simulink model "ex2busStability_sim"  (R2014b)
settings: Solver=ode45  SolverMode=SingleTasking  StartTime=0  StopTime=10  MaxStep=0.001  RelTol=1e-06
values from neighbouring files (symbols this model uses):
  A = full(A)    [ex3busPV.m]
  B = full(B)    [ex3busPV.m]
  C = full(C)    [ex3busPV.m]    (also in ex_get_started_here.m = 5e-07; pv_dq.m = 4.01652892562e-06)
  cur_dq0_op = 2^0.5*[-iopx; iopx; -iopy; iopy; 0; 0]    [ex2busStability.m]
  D = full(D)    [ex3busPV.m]
  Kd = KD_GAIN_CNST*J*ws    [ex14busSGandPV.m]    (also in ex2busStability.m = 24000; ex7busLongLine.m; ex9busSG.m; exDroopA.m)
  lamda = (2^0.5) * Vgmag/ws    (= 45.916132124)    [ex2busStability.m]    (also in ex9busSG.m = (2^0.5) * Vn_gens/ws)
  Pm_op = 3*Pg    (= 600000)    [ex2busStability.m]
  poles_2Jws = poles./(2*J*ws)    [ex14busSGandPV.m]    (also in ex2busStability.m = poles./(2*ws*J); ex7busLongLine.m; ex9busSG.m = poles./(2*ws*J); exDroopA.m)
  step_size = 30e3    (= 30000)    [ex2busStability.m]    (also in exDroopB.m = 0)
  step_time = 9    [ex2busStability.m]    (also in ex3busPV.m = 0.05; exDroopB.m = 10; exLongLinePV.m = 1; syncMachVsSwing.m = 5)
  V1mag = 10e3    (= 10000)    [ex2busStability.m]
  vol_dq0_op = 2^0.5*[V1mag; vopx; 0; vopy; 0; 0]    [ex2busStability.m]
  ws = 2*pi*50    (= 314.159265359)    [ex14busSGandPV.m]    (also in ex2busStability.m; ex3busPV.m; ex7busLongLine.m; ex9busSG.m)
undefined symbols (not defined in the file or in its folder): Anet, Bnet, Cnet, Dnet, full
settings Model: Creator=COPEC  LastModifiedBy=Juri
settings OptimizationCC: BlockReduction=off  BooleanDataType=off
settings DebuggingCC: SaveWithParameterizedLinksMsg=none  UnderspecifiedInitializationDetection=Classic  MergeDetectMultiDrivingBlocksExec=none  SignalResolutionControl=TryResolveAllWithWarning  SolverPrmCheckMsg=none  FrameProcessingCompatibilityMsg=error
settings HardwareCC: TargetUnknown=on

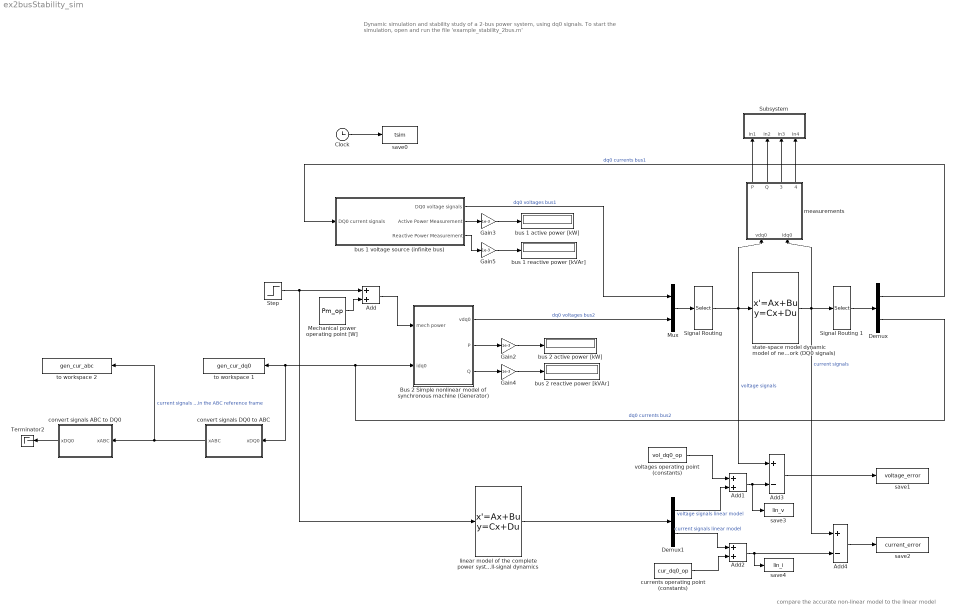
== system ex2busStability_sim ==
  note: Dynamic simulation and stability study of a 2-bus power system,
      | using dq0 signals.
      |
      | To start the simulation, open and run the file
      | 'example_stability_2bus.m'
  note: compare the accurate non-linear model to the linear model
  Add : Sum
  Add1 : Sum
  Add2 : Sum
  Add3 : Sum  Inputs=+-
  Add4 : Sum  Inputs=+-
  Bus 2 Simple nonlinear model of synchronous machine (Generator) : Subsystem
  Clock : Clock
  Demux : Demux  Outputs=2
  Demux1 : Demux  Outputs=2
  Gain{2..5} (4 alike) : Gain  Gain=1e-3
  Mechanical power operating point [W] : Constant  Value=Pm_op
  Mux : Mux  Inputs=2
  "Signal Routing " : Selector  InputPortWidth=6  IndexOptions=Index vector (dialog)  Indices=[1 4 2 5 3 6]  OutputSizes=1
  Signal Routing 1 : Selector  InputPortWidth=6  IndexOptions=Index vector (dialog)  Indices=[1 3 5 2 4 6]  OutputSizes=1
  Step : Step  Time=step_time  After=step_size  SampleTime=0
  Subsystem : Subsystem
  Terminator2 : Terminator
  bus 1 voltage source (infinite bus) : Subsystem
  bus 1 active power [kW] : Display
  bus 1 reactive power [kVAr] : Display
  bus 2 active power [kW] : Display
  bus 2 reactive power [kVAr] : Display
  convert signals ABC to DQ0 : Subsystem
  convert signals DQ0 to ABC : Subsystem
  currents operating point (constants) : Constant  Value=cur_dq0_op
  "linear model of the complete power system (network + generator) this state-space model represents the system small-signal dynamics " : StateSpace  A=full(A)  B=full(B)  C=full(C)  D=full(D)  X0=0
  measurements : Subsystem
  save0 : ToWorkspace  VariableName=tsim  SampleTime=-1
  save1 : ToWorkspace  VariableName=voltage_error  SampleTime=-1
  save2 : ToWorkspace  VariableName=current_error  SampleTime=-1
  save3 : ToWorkspace  VariableName=lin_v  SampleTime=-1
  save4 : ToWorkspace  VariableName=lin_i  SampleTime=-1
  state-space model dynamic model of network (DQ0 signals) : StateSpace  A=full(Anet)  B=full(Bnet)  C=full(Cnet)  D=full(Dnet)  X0=0
  to workspace 1 : ToWorkspace  VariableName=gen_cur_dq0  SampleTime=-1
  to workspace 2 : ToWorkspace  VariableName=gen_cur_abc  SampleTime=-1
  voltages operating point (constants) : Constant  Value=vol_dq0_op
  wires:
  Clock/1 -> save0/1
  Gain2/1 -> bus 2 active power [kW]/1
  Gain4/1 -> bus 2 reactive power [kVAr]/1
  Mechanical power operating point [W]/1 -> Add/2
  Mux/1 -> "Signal Routing "/1
  Signal Routing 1/1 -> Demux/1
  Bus 2 Simple nonlinear model of synchronous machine (Generator)/2(P) -> Gain2/1
  Bus 2 Simple nonlinear model of synchronous machine (Generator)/3(Q) -> Gain4/1
  "Signal Routing "/1 -> Add3/1, state-space model dynamic model of network (DQ0 signals)/1, measurements/1(vdq0)  "voltage signals"
  bus 1 voltage source (infinite bus)/1(DQ0 voltage signals) -> Mux/1  "dq0 voltages bus1"
  Bus 2 Simple nonlinear model of synchronous machine (Generator)/1(vdq0) -> Mux/2  "dq0 voltages bus2"
  Demux/1 -> bus 1 voltage source (infinite bus)/1(DQ0 current signals)  "dq0 currents bus1"
  Demux/2 -> to workspace 1/1, convert signals DQ0 to ABC/1(xDQ0), Bus 2 Simple nonlinear model of synchronous machine (Generator)/2(idq0)  "dq0 currents bus2"
  state-space model dynamic model of network (DQ0 signals)/1 -> Add4/1, measurements/2(idq0), Signal Routing 1/1  "current signals"
  convert signals DQ0 to ABC/1(xABC) -> to workspace 2/1, convert signals ABC to DQ0/1(xABC)  "current signals in the ABC reference frame"
  convert signals ABC to DQ0/1(xDQ0) -> Terminator2/1
  bus 1 voltage source (infinite bus)/2(Active Power Measurement) -> Gain3/1
  bus 1 voltage source (infinite bus)/3("Reactive Power Measurement ") -> Gain5/1
  Gain3/1 -> bus 1 active power [kW]/1
  Gain5/1 -> bus 1 reactive power [kVAr]/1
  Add/1 -> Bus 2 Simple nonlinear model of synchronous machine (Generator)/1(mech power)
  Step/1 -> "linear model of the complete power system (network + generator) this state-space model represents the system small-signal dynamics "/1, Add/1
  "linear model of the complete power system (network + generator) this state-space model represents the system small-signal dynamics "/1 -> Demux1/1
  Demux1/1 -> Add1/2  "voltage signals linear model"
  Demux1/2 -> Add2/1  "current signals linear model"
  voltages operating point (constants)/1 -> Add1/1
  currents operating point (constants)/1 -> Add2/2
  Add1/1 -> save3/1, Add3/2
  Add2/1 -> save4/1, Add4/2
  Add3/1 -> save1/1
  Add4/1 -> save2/1
  measurements/1(P) -> Subsystem/1(In1)
  measurements/2(Q) -> Subsystem/2(In2)
  measurements/3(Vm_RMS) -> Subsystem/3(In3)
  measurements/4(Vph_deg) -> Subsystem/4(In4)

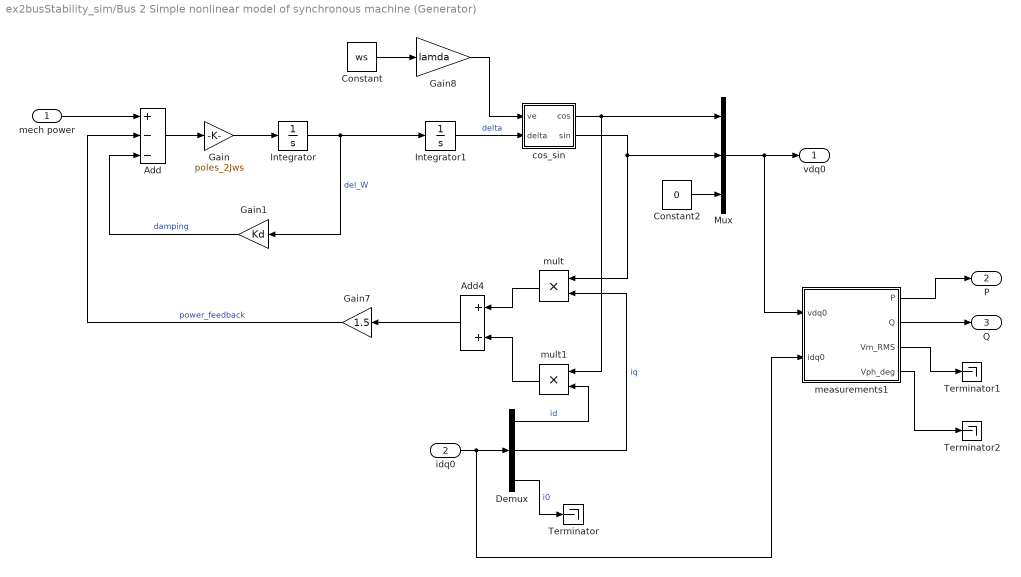
== system ex2busStability_sim/Bus 2 Simple nonlinear model of synchronous machine (Generator) ==
  mech power : Inport
  idq0 : Inport  Port=2
  Add : Sum  Inputs=+--
  Add4 : Sum
  Constant : Constant  Value=ws
  Constant2 : Constant  Value=0
  Demux : Demux  Outputs=3
  Gain : Gain  Gain=poles_2Jws
  Gain1 : Gain  Gain=Kd
  Gain7 : Gain  Gain=1.5
  Gain8 : Gain  Gain=lamda
  Integrator : Integrator
  Integrator1 : Integrator
  Mux : Mux  Inputs=3
  Terminator : Terminator
  Terminator1 : Terminator
  Terminator2 : Terminator
  cos_sin : Subsystem
  measurements1 : Subsystem
  mult : Product  Inputs=**
  mult1 : Product  Inputs=**
  vdq0 : Outport
  P : Outport  Port=2
  Q : Outport  Port=3
  wires:
  mech power/1 -> Add/1
  Add/1 -> Gain/1
  Gain/1 -> Integrator/1
  Integrator/1 -> Gain1/1, Integrator1/1  "del_W"
  Integrator1/1 -> cos_sin/2(delta)  "delta"
  Gain1/1 -> Add/3  "damping"
  Demux/3 -> Terminator/1  "i0"
  cos_sin/1(cos) -> mult1/1, Mux/1
  cos_sin/2(sin) -> mult/1, Mux/2
  mult/1 -> Add4/1
  mult1/1 -> Add4/2
  Add4/1 -> Gain7/1
  Gain7/1 -> Add/2  "power_feedback"
  idq0/1 -> measurements1/2(idq0), Demux/1
  Mux/1 -> measurements1/1(vdq0), vdq0/1
  Constant/1 -> Gain8/1
  Gain8/1 -> cos_sin/1(ve)
  Constant2/1 -> Mux/3
  Demux/1 -> mult1/2  "id"
  Demux/2 -> mult/2  "iq"
  measurements1/1(P) -> P/1
  measurements1/2(Q) -> Q/1
  measurements1/3(Vm_RMS) -> Terminator1/1
  measurements1/4(Vph_deg) -> Terminator2/1

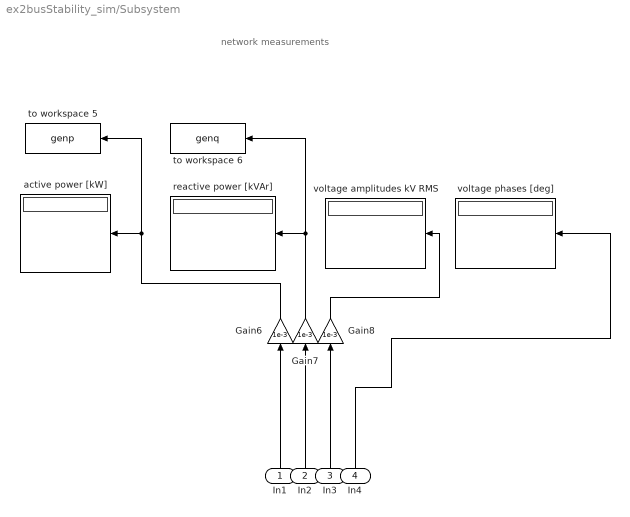
== system ex2busStability_sim/Subsystem ==
  note: network measurements
  In1 : Inport
  In2 : Inport  Port=2
  In3 : Inport  Port=3
  In4 : Inport  Port=4
  Gain6 : Gain  Gain=1e-3
  Gain7 : Gain  Gain=1e-3
  Gain8 : Gain  Gain=1e-3
  active power [kW] : Display
  reactive power [kVAr] : Display
  to workspace 5 : ToWorkspace  VariableName=genp  SampleTime=-1
  to workspace 6 : ToWorkspace  VariableName=genq  SampleTime=-1
  "voltage amplitudes kV RMS " : Display
  voltage phases [deg] : Display
  wires:
  Gain6/1 -> to workspace 5/1, active power [kW]/1
  In1/1 -> Gain6/1
  In3/1 -> Gain8/1
  In2/1 -> Gain7/1
  Gain8/1 -> "voltage amplitudes kV RMS "/1
  Gain7/1 -> to workspace 6/1, reactive power [kVAr]/1
  In4/1 -> voltage phases [deg]/1

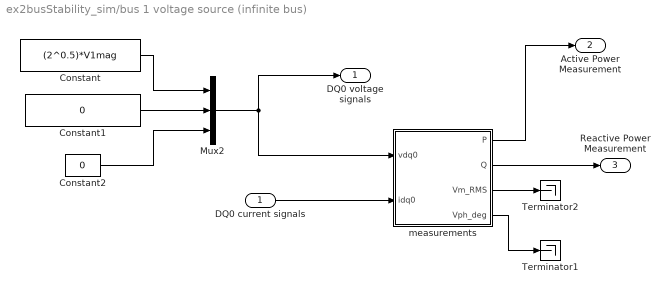
== system ex2busStability_sim/bus 1 voltage source (infinite bus) ==
  DQ0 current signals : Inport
  Constant : Constant  Value=(2^0.5)*V1mag
  Constant1 : Constant  Value=0
  Constant2 : Constant  Value=0
  Mux2 : Mux  Inputs=3
  Terminator1 : Terminator
  Terminator2 : Terminator
  measurements : Subsystem
  DQ0 voltage signals : Outport
  Active Power Measurement : Outport  Port=2
  "Reactive Power Measurement " : Outport  Port=3
  wires:
  Constant/1 -> Mux2/1
  Constant1/1 -> Mux2/2
  Constant2/1 -> Mux2/3
  Mux2/1 -> measurements/1(vdq0), DQ0 voltage signals/1
  DQ0 current signals/1 -> measurements/2(idq0)
  measurements/1(P) -> Active Power Measurement/1
  measurements/2(Q) -> "Reactive Power Measurement "/1
  measurements/3(Vm_RMS) -> Terminator2/1
  measurements/4(Vph_deg) -> Terminator1/1

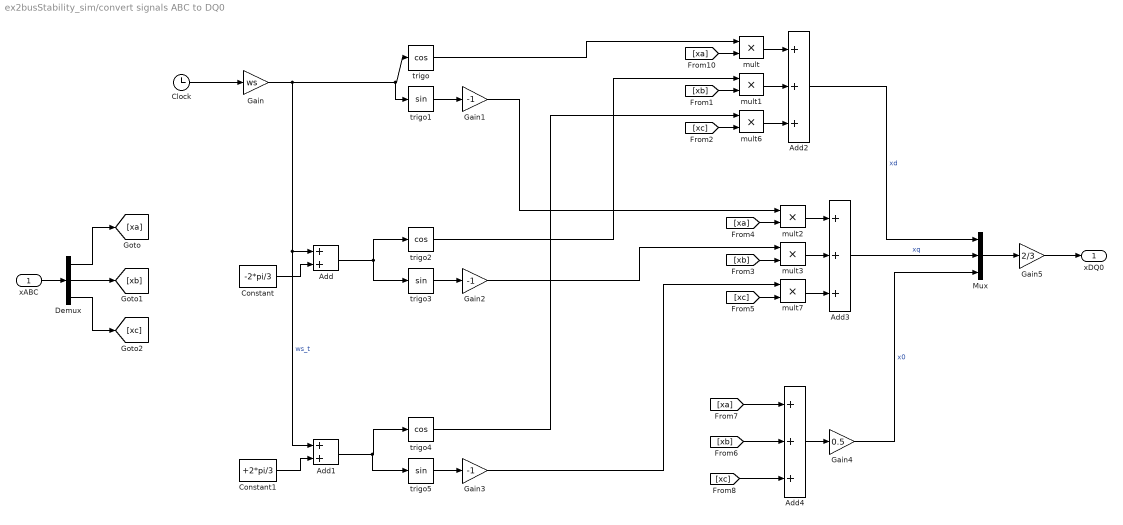
== system ex2busStability_sim/convert signals ABC to DQ0 ==
  xABC : Inport
  Add : Sum
  Add1 : Sum
  Add2 : Sum  Inputs=+++
  Add3 : Sum  Inputs=+++
  Add4 : Sum  Inputs=+++
  Clock : Clock
  Constant : Constant  Value=-2*pi/3
  Constant1 : Constant  Value=+2*pi/3
  Demux : Demux  Outputs=3
  Gain : Gain  Gain=ws
  Gain1 : Gain  Gain=-1
  Gain2 : Gain  Gain=-1
  Gain3 : Gain  Gain=-1
  Gain4 : Gain  Gain=0.5
  Gain5 : Gain  Gain=2/3
  Mux : Mux  Inputs=3
  mult{,1..3,6..7} (6 alike) : Product  Inputs=**
  trigo : Trigonometry  Operator=cos
  trigo1 : Trigonometry
  trigo2 : Trigonometry  Operator=cos
  trigo3 : Trigonometry
  trigo4 : Trigonometry  Operator=cos
  trigo5 : Trigonometry
  xDQ0 : Outport
  wires:
  Gain5/1 -> xDQ0/1
  Mux/1 -> Gain5/1
  Gain3/1 -> mult7/1
  Gain2/1 -> mult3/1
  Gain1/1 -> mult2/1
  [xc] -> Add4/3
  [xb] -> Add4/2
  [xa] -> Add4/1
  Add4/1 -> Gain4/1
  mult7/1 -> Add3/3
  [xc] -> mult7/2
  [xb] -> mult3/2
  [xa] -> mult2/2
  trigo4/1 -> mult6/1
  mult6/1 -> Add2/3
  [xc] -> mult6/2
  trigo2/1 -> mult1/1
  trigo/1 -> mult/1
  Gain4/1 -> Mux/3  "x0"
  Add3/1 -> Mux/2  "xq"
  Add2/1 -> Mux/1  "xd"
  mult3/1 -> Add3/2
  mult2/1 -> Add3/1
  [xb] -> mult1/2
  [xa] -> mult/2
  mult1/1 -> Add2/2
  mult/1 -> Add2/1
  Demux/3 -> [xc]
  Demux/2 -> [xb]
  Demux/1 -> [xa]
  xABC/1 -> Demux/1
  Add1/1 -> trigo4/1, trigo5/1
  trigo5/1 -> Gain3/1
  Add/1 -> trigo3/1, trigo2/1
  trigo3/1 -> Gain2/1
  trigo1/1 -> Gain1/1
  Constant1/1 -> Add1/2
  Constant/1 -> Add/2
  Gain/1 -> Add/1, Add1/1, trigo/1, trigo1/1  "ws_t"
  Clock/1 -> Gain/1

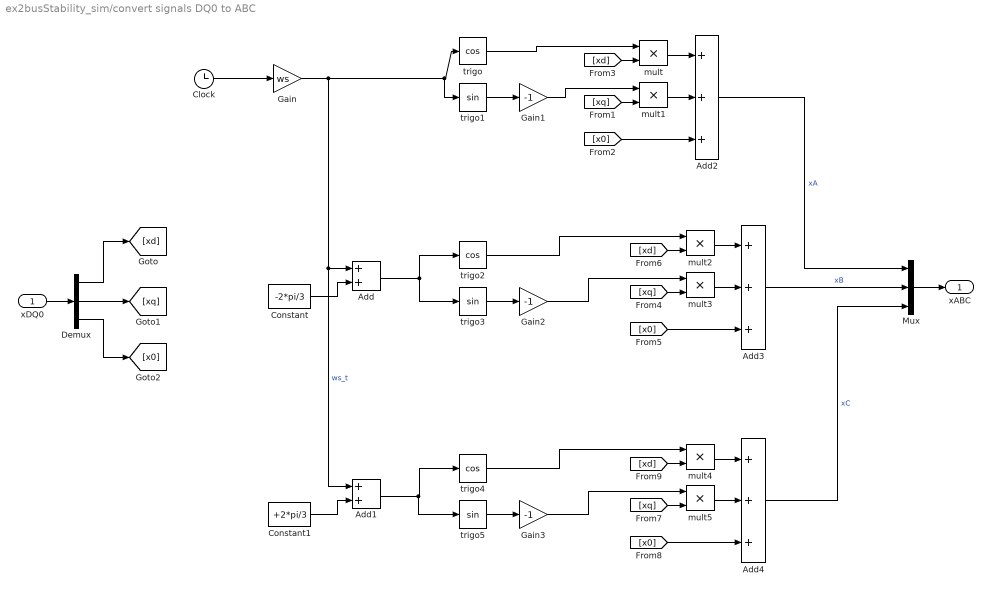
== system ex2busStability_sim/convert signals DQ0 to ABC ==
  xDQ0 : Inport
  Add : Sum
  Add1 : Sum
  Add2 : Sum  Inputs=+++
  Add3 : Sum  Inputs=+++
  Add4 : Sum  Inputs=+++
  Clock : Clock
  Constant : Constant  Value=-2*pi/3
  Constant1 : Constant  Value=+2*pi/3
  Demux : Demux  Outputs=3
  Gain : Gain  Gain=ws
  Gain1 : Gain  Gain=-1
  Gain2 : Gain  Gain=-1
  Gain3 : Gain  Gain=-1
  Mux : Mux  Inputs=3
  mult{,1..5} (6 alike) : Product  Inputs=**
  trigo : Trigonometry  Operator=cos
  trigo1 : Trigonometry
  trigo2 : Trigonometry  Operator=cos
  trigo3 : Trigonometry
  trigo4 : Trigonometry  Operator=cos
  trigo5 : Trigonometry
  xABC : Outport
  wires:
  Clock/1 -> Gain/1
  Gain/1 -> trigo1/1, trigo/1, Add1/1, Add/1  "ws_t"
  Constant/1 -> Add/2
  Constant1/1 -> Add1/2
  trigo1/1 -> Gain1/1
  trigo3/1 -> Gain2/1
  Add/1 -> trigo2/1, trigo3/1
  trigo5/1 -> Gain3/1
  Add1/1 -> trigo5/1, trigo4/1
  xDQ0/1 -> Demux/1
  Demux/1 -> [xd]
  Demux/2 -> [xq]
  Demux/3 -> [x0]
  Mux/1 -> xABC/1
  mult/1 -> Add2/1
  mult1/1 -> Add2/2
  [xd] -> mult/2
  [xq] -> mult1/2
  [x0] -> Add2/3
  mult2/1 -> Add3/1
  mult3/1 -> Add3/2
  [xd] -> mult2/2
  [xq] -> mult3/2
  [x0] -> Add3/3
  mult4/1 -> Add4/1
  mult5/1 -> Add4/2
  [xd] -> mult4/2
  [xq] -> mult5/2
  [x0] -> Add4/3
  trigo/1 -> mult/1
  Gain1/1 -> mult1/1
  trigo2/1 -> mult2/1
  Gain2/1 -> mult3/1
  trigo4/1 -> mult4/1
  Gain3/1 -> mult5/1
  Add2/1 -> Mux/1  "xA"
  Add3/1 -> Mux/2  "xB"
  Add4/1 -> Mux/3  "xC"

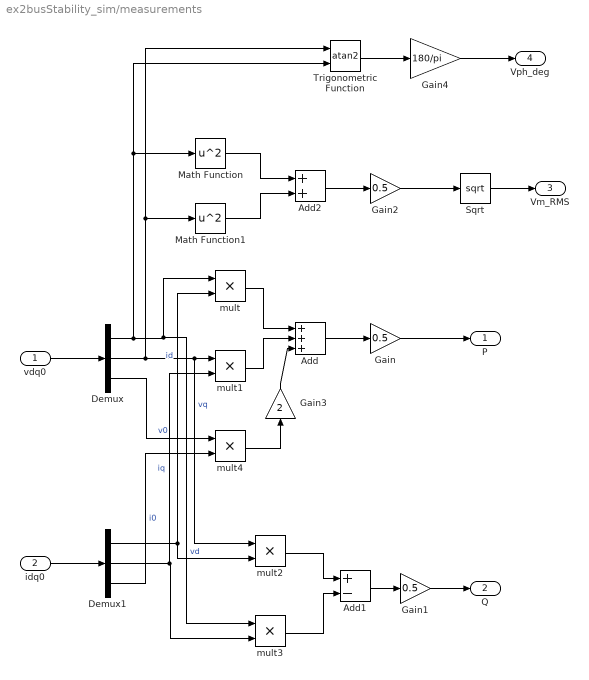
== system ex2busStability_sim/measurements ==
  vdq0 : Inport
  idq0 : Inport  Port=2
  Add : Sum  Inputs=+++
  Add1 : Sum  Inputs=+-
  Add2 : Sum
  Demux : Demux  Outputs=3
  Demux1 : Demux  Outputs=3
  Gain : Gain  Gain=0.5
  Gain1 : Gain  Gain=0.5
  Gain2 : Gain  Gain=0.5
  Gain3 : Gain  Gain=2
  Gain4 : Gain  Gain=180/pi
  Math Function : Math  Operator=square  SaturateOnIntegerOverflow=on
  Math Function1 : Math  Operator=square  SaturateOnIntegerOverflow=on
  Sqrt : Sqrt  SaturateOnIntegerOverflow=on
  Trigonometric Function : Trigonometry  Operator=atan2
  mult{,1..4} (5 alike) : Product  Inputs=**
  P : Outport
  Q : Outport  Port=2
  Vm_RMS : Outport  Port=3
  Vph_deg : Outport  Port=4
  wires:
  idq0/1 -> Demux1/1
  vdq0/1 -> Demux/1
  Demux/1 -> Math Function/1, Trigonometric Function/2, mult3/1, mult/1  "vd"
  Demux/2 -> Trigonometric Function/1, Math Function1/1, mult2/1, mult1/1  "vq"
  Demux1/1 -> mult/2, mult2/2  "id"
  Demux1/2 -> mult3/2, mult1/2  "iq"
  Demux/3 -> mult4/1  "v0"
  Demux1/3 -> mult4/2  "i0"
  mult/1 -> Add/1
  mult1/1 -> Add/2
  Add/1 -> Gain/1
  mult2/1 -> Add1/1
  mult3/1 -> Add1/2
  Add1/1 -> Gain1/1
  Sqrt/1 -> Vm_RMS/1
  Math Function/1 -> Add2/1
  Math Function1/1 -> Add2/2
  Add2/1 -> Gain2/1
  Gain2/1 -> Sqrt/1
  Gain/1 -> P/1
  Gain1/1 -> Q/1
  mult4/1 -> Gain3/1
  Gain3/1 -> Add/3
  Trigonometric Function/1 -> Gain4/1
  Gain4/1 -> Vph_deg/1

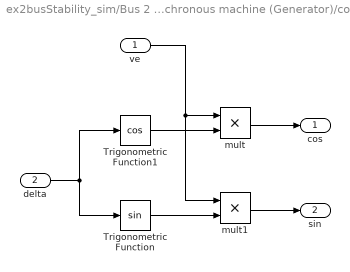
== system ex2busStability_sim/Bus 2 Simple nonlinear model of synchronous machine (Generator)/cos_sin ==
  ve : Inport
  delta : Inport  Port=2
  Trigonometric Function : Trigonometry
  Trigonometric Function1 : Trigonometry  Operator=cos
  mult : Product  Inputs=**
  mult1 : Product  Inputs=**
  cos : Outport
  sin : Outport  Port=2
  wires:
  delta/1 -> Trigonometric Function/1, Trigonometric Function1/1
  Trigonometric Function1/1 -> mult/2
  ve/1 -> mult1/1, mult/1
  Trigonometric Function/1 -> mult1/2
  mult/1 -> cos/1
  mult1/1 -> sin/1

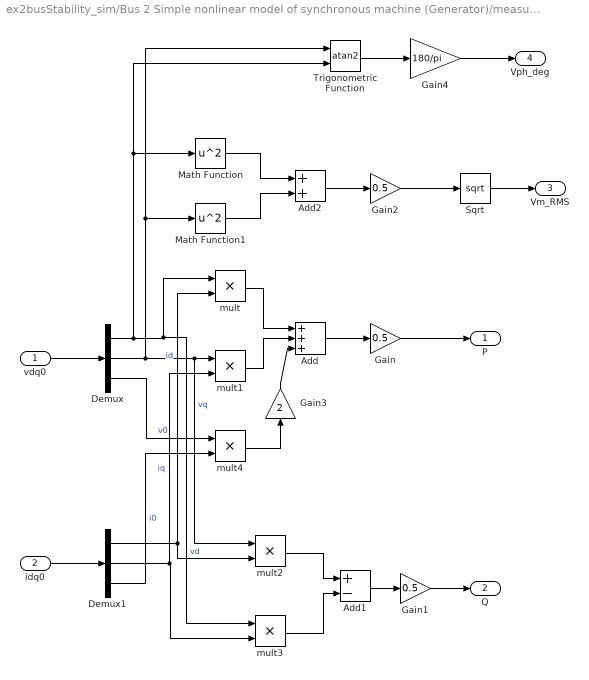
== system ex2busStability_sim/Bus 2 Simple nonlinear model of synchronous machine (Generator)/measurements1 ==
  vdq0 : Inport
  idq0 : Inport  Port=2
  Add : Sum  Inputs=+++
  Add1 : Sum  Inputs=+-
  Add2 : Sum
  Demux : Demux  Outputs=3
  Demux1 : Demux  Outputs=3
  Gain : Gain  Gain=0.5
  Gain1 : Gain  Gain=0.5
  Gain2 : Gain  Gain=0.5
  Gain3 : Gain  Gain=2
  Gain4 : Gain  Gain=180/pi
  Math Function : Math  Operator=square  SaturateOnIntegerOverflow=on
  Math Function1 : Math  Operator=square  SaturateOnIntegerOverflow=on
  Sqrt : Sqrt  SaturateOnIntegerOverflow=on
  Trigonometric Function : Trigonometry  Operator=atan2
  mult{,1..4} (5 alike) : Product  Inputs=**
  P : Outport
  Q : Outport  Port=2
  Vm_RMS : Outport  Port=3
  Vph_deg : Outport  Port=4
  wires:
  idq0/1 -> Demux1/1
  vdq0/1 -> Demux/1
  Demux/1 -> Math Function/1, Trigonometric Function/2, mult3/1, mult/1  "vd"
  Demux/2 -> Trigonometric Function/1, Math Function1/1, mult2/1, mult1/1  "vq"
  Demux1/1 -> mult/2, mult2/2  "id"
  Demux1/2 -> mult3/2, mult1/2  "iq"
  Demux/3 -> mult4/1  "v0"
  Demux1/3 -> mult4/2  "i0"
  mult/1 -> Add/1
  mult1/1 -> Add/2
  Add/1 -> Gain/1
  mult2/1 -> Add1/1
  mult3/1 -> Add1/2
  Add1/1 -> Gain1/1
  Sqrt/1 -> Vm_RMS/1
  Math Function/1 -> Add2/1
  Math Function1/1 -> Add2/2
  Add2/1 -> Gain2/1
  Gain2/1 -> Sqrt/1
  Gain/1 -> P/1
  Gain1/1 -> Q/1
  mult4/1 -> Gain3/1
  Gain3/1 -> Add/3
  Trigonometric Function/1 -> Gain4/1
  Gain4/1 -> Vph_deg/1

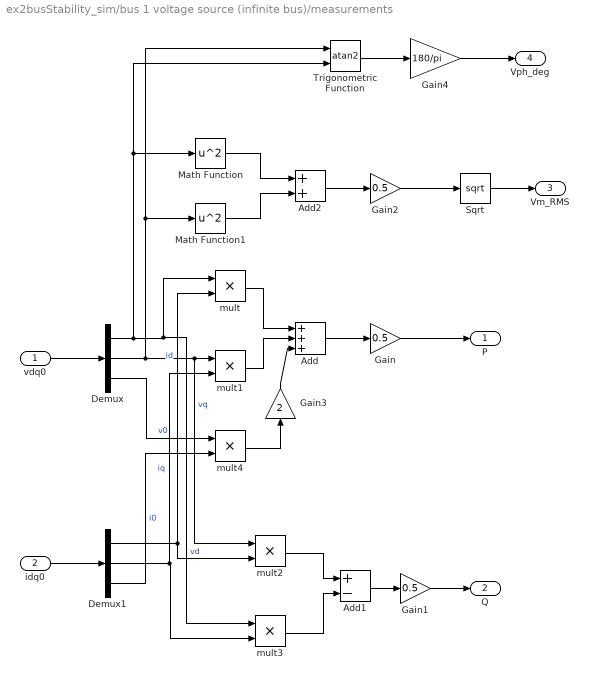
== system ex2busStability_sim/bus 1 voltage source (infinite bus)/measurements ==
  vdq0 : Inport
  idq0 : Inport  Port=2
  Add : Sum  Inputs=+++
  Add1 : Sum  Inputs=+-
  Add2 : Sum
  Demux : Demux  Outputs=3
  Demux1 : Demux  Outputs=3
  Gain : Gain  Gain=0.5
  Gain1 : Gain  Gain=0.5
  Gain2 : Gain  Gain=0.5
  Gain3 : Gain  Gain=2
  Gain4 : Gain  Gain=180/pi
  Math Function : Math  Operator=square  SaturateOnIntegerOverflow=on
  Math Function1 : Math  Operator=square  SaturateOnIntegerOverflow=on
  Sqrt : Sqrt  SaturateOnIntegerOverflow=on
  Trigonometric Function : Trigonometry  Operator=atan2
  mult{,1..4} (5 alike) : Product  Inputs=**
  P : Outport
  Q : Outport  Port=2
  Vm_RMS : Outport  Port=3
  Vph_deg : Outport  Port=4
  wires:
  idq0/1 -> Demux1/1
  vdq0/1 -> Demux/1
  Demux/1 -> Math Function/1, Trigonometric Function/2, mult3/1, mult/1  "vd"
  Demux/2 -> Trigonometric Function/1, Math Function1/1, mult2/1, mult1/1  "vq"
  Demux1/1 -> mult/2, mult2/2  "id"
  Demux1/2 -> mult3/2, mult1/2  "iq"
  Demux/3 -> mult4/1  "v0"
  Demux1/3 -> mult4/2  "i0"
  mult/1 -> Add/1
  mult1/1 -> Add/2
  Add/1 -> Gain/1
  mult2/1 -> Add1/1
  mult3/1 -> Add1/2
  Add1/1 -> Gain1/1
  Sqrt/1 -> Vm_RMS/1
  Math Function/1 -> Add2/1
  Math Function1/1 -> Add2/2
  Add2/1 -> Gain2/1
  Gain2/1 -> Sqrt/1
  Gain/1 -> P/1
  Gain1/1 -> Q/1
  mult4/1 -> Gain3/1
  Gain3/1 -> Add/3
  Trigonometric Function/1 -> Gain4/1
  Gain4/1 -> Vph_deg/1
